simulink model "lee_pos_controller"  (R2023a)
settings: Solver=VariableStepAuto  StartTime=0.0  StopTime=10.0  RelTol=1e-3
undefined symbols (not defined in the file): g, K_v, K_x, mass_total
settings Model: Creator=jonas  LastModifiedBy=jonas

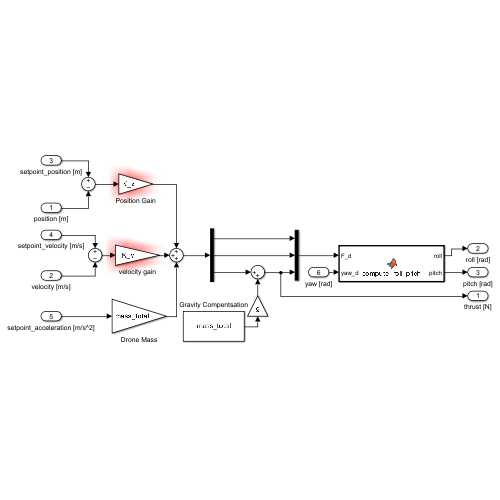
[thumbnail: Simulink's stored preview of the top-level diagram]
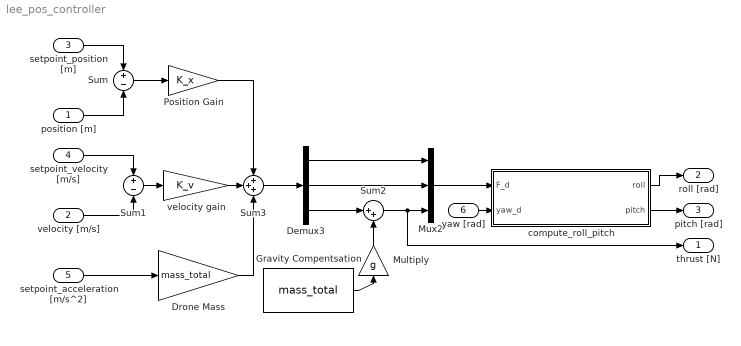
== system lee_pos_controller ==
  position [m] : Inport
  velocity [m/s] : Inport  Port=2
  setpoint_position [m] : Inport  Port=3
  setpoint_velocity [m/s] : Inport  Port=4
  setpoint_acceleration [m/s^2] : Inport  Port=5
  yaw [rad] : Inport  Port=6
  Demux3 : Demux  Outputs=3
  Drone Mass : Gain  Gain=mass_total
  Gravity Compentsation : Constant  Value=mass_total  VectorParams1D=off
  Multiply : Gain  Gain=g
  Mux2 : Mux  Inputs=3
  Position Gain : Gain  Gain=K_x
  Sum : Sum  Inputs=+|-
  Sum1 : Sum  Inputs=+|-
  Sum2 : Sum  Inputs=|++
  Sum3 : Sum  Inputs=+++
  compute_roll_pitch : MATLAB Function  TreatAsAtomicUnit=on
  velocity gain : Gain  Gain=K_v
  thrust [N] : Outport
  roll [rad] : Outport  Port=2
  pitch [rad] : Outport  Port=3
  wires:
  Position Gain/1 -> Sum3/1
  Sum1/1 -> velocity gain/1
  setpoint_acceleration [m/s^2]/1 -> Drone Mass/1
  velocity gain/1 -> Sum3/2
  position [m]/1 -> Sum/2
  Demux3/1 -> Mux2/1
  yaw [rad]/1 -> compute_roll_pitch/2(yaw_d)
  setpoint_velocity [m/s]/1 -> Sum1/1
  compute_roll_pitch/2(pitch) -> pitch [rad]/1
  Multiply/1 -> Sum2/2
  Demux3/2 -> Mux2/2
  compute_roll_pitch/1(roll) -> roll [rad]/1
  Sum3/1 -> Demux3/1
  Mux2/1 -> compute_roll_pitch/1(F_d)
  Gravity Compentsation/1 -> Multiply/1
  setpoint_position [m]/1 -> Sum/1
  Demux3/3 -> Sum2/1
  velocity [m/s]/1 -> Sum1/2
  Drone Mass/1 -> Sum3/3
  Sum/1 -> Position Gain/1
  Sum2/1 -> thrust [N]/1, Mux2/3

== matlab function lee_pos_controller/compute_roll_pitch ==
  data: F_d input; roll output; yaw_d input; pitch output
function [roll, pitch] = compute_roll_pitch(F_d, yaw_d)

yaw_dt = yaw_d + pi/2;
uyt = [cos(yaw_dt); sin(yaw_dt); 0];
uz = F_d/norm(F_d);
ux = cross(uyt, uz);
uy = cross(uz, ux);

attitude = rotm2eul([ux uy uz], 'ZYX');

roll = attitude(3);
pitch = attitude(2);
